simulink model "controlador_discreto"  (R2023b)
settings: Solver=FixedStepAuto  StartTime=0.0  StopTime=25  FixedStep=0.001  RelTol=1e-3
undefined symbols (not defined in the file): b_cx, b_cy, b_hb, b_hEb, b_hwu, b_t, b_tb, b_tw, bh_eq, bh_eq_prima, bt_eq, CI, ddx_t_lim, ddy_h_lim, DiscIntNeverNeededParam, dx_t_lim, dy_h_lim, g, H_c, H_SS, i_h, i_t, Jh_eq, Jh_eq_aux, Jt_eq, K_cy, K_hwu, K_tw, Kd_h, Kd_t, Ki_h, Ki_t, Kp_h, Kp_t, L_h0, M_s, m_t, r_hd, r_td, T_hb_max, T_hEb_max, T_hm_max, T_s1, T_s2, T_tb_max, T_tm_max, tau_hm, tau_tm, W_c, x_t_lim, y_c, y_h_lim, Y_t0
libraries: simulink x19, sldrtlib x1, simulink_extras x1
(part 2 of 2)

== stateflow chart controlador_discreto/Nivel 1 ==
  state Toma_carga_manual [commented out]
  state Mapeo_entradas_digitales
    accion_muelle = inputs(1);
    n_muelle = inputs(2);
    p_ini = inputs(3);
    p_fin = inputs(4);
  state Accion_carga_automatico
    state Precalculos
      % Calculos para realizar las maniobras pertinentes
      y_max = max(y_c(1:p_fin));
      %CI(3) = y_max;
      v_act = 10
    state Prueba
      carro_cons = [0 0]
      izaje_cons = [0 0]
      [carro_cons, izaje_cons] = consigna_en_muelle(T_s1, W_c, set_param_lim, n_muelle, y_max , 0, H_SS, 0, 0)
    state Toma_carga_muelle_automatico
      % Se toma carga desde posicion en muelle y se lleva al barco
      % -------------
      entry:
      [carro_cons, izaje_cons] = consigna_en_muelle(T_s1, W_c, set_param_lim, n_muelle, y_max , 0, H_SS, 0, 0);
      idx_t = 1; idx_h = 1;
      flag = 1; % CAMBIAR !!!!
      % -------------
      during:
      % Carro
      x_t = carro_cons(idx_t, 1);
      dx_t = carro_cons(idx_t, 2);
      % Izaje
      y_h = izaje_cons(idx_h, 1);
      dy_h = izaje_cons(idx_h, 2);
      if idx_t  ~=  length(carro_cons)
      idx_t = idx_t + 1;
      end
      if idx_h  ~=  length(izaje_cons)
      idx_h = idx_h + 1;
      end
      if idx_t == length(carro_cons) && idx_h == length(izaje_cons)
      flag = 1;
      end
    state Deja_carga_barco [commented out]
      % Se entra con v_t y deja carga en barco
      % -------------
      entry:
      %[carro_cons, izaje_cons] = consigna_en_barco(T_s1, W_c, H_c, y_c, set_param_lim, p_ini, p_fin, H_SS, 0, 0, 1);
      [carro_cons, izaje_cons] = consigna_en_barco(T_s1, W_c, H_c, [1 2 3], set_param_lim, 0, 1, 0.5, 0, 0, 1);
      idx_t = 1; idx_h = 1;
      flag = 0;
      % -------------
      during:
      % Carro
      x_t = carro_cons(idx_t, 1);
      dx_t = carro_cons(idx_t, 2);
      % Izaje
      y_h = izaje_cons(idx_h, 1);
      dy_h = izaje_cons(idx_h, 2);
      if idx_t  ~=  length(carro_cons)
      idx_t = idx_t + 1;
      end
      if idx_h  ~=  length(izaje_cons)
      idx_h = idx_h + 1;
      end
      if idx_t == length(carro_cons) && idx_h == length(izaje_cons)
      flag = 1;
      end
    (default) -> Precalculos
    Toma_carga_muelle_automatico -> Prueba : [flag == 1]
    Precalculos -> Toma_carga_muelle_automatico : [v_act == 10]
    Toma_carga_muelle_automatico -> Deja_carga_barco [commented out] : [flag == 1]
        | {
        | carro_cons = [0 0],
        | izaje_cons = [0 0]
        | }
  state IDLE
    entry:
    set_param_lim = [dx_t_lim ddx_t_lim dy_h_lim(1) ddy_h_lim];
    altura_izaje = 15;
    v_act = 0;
  state Deja_carga_muelle_automatico
    % Se deja carga en el muelle (especificando numero de muelle), entrando al mismo a velocidad v_act de carro
    % ------
    entry:
    [carro_cons, izaje_cons] = consigna_en_muelle(T_s1, W_c, set_param_lim, n_muelle, altura_izaje, 1, H_SS, v_act);
    idx_t = 1; idx_h = 1;
    flag = 0;
    % -------
    during:
    % Carro
    x_t = carro_cons(idx_t, 1);
    dx_t = carro_cons(idx_t, 2);
    % Izaje
    y_h = izaje_cons(idx_h, 1);
    dy_h = izaje_cons(idx_h, 2);
    if idx_t  ~=  length(carro_cons)
    idx_t = idx_t + 1;
    end
    if idx_h  ~=  length(izaje_cons)
    idx_h = idx_h + 1;
    end
    if idx_t == length(carro_cons) && idx_h == length(izaje_cons)
    flag = 1;
    end
  (default) -> Mapeo_entradas_digitales
  Mapeo_entradas_digitales -> IDLE
  IDLE -> Accion_carga_automatico [order 1] : [accion_muelle == 0]
  IDLE -> Deja_carga_muelle_automatico [order 2] : [accion_muelle == 1]
  data: inputs input size=4; T_s1 parameter; carro_cons local size=[10000; 10000] =[CI(1) CI(2)]; izaje_cons local size=[10000; 10000] =[CI(3) CI(4)]; W_c parameter; ddx_t_lim parameter; ddy_h_lim parameter; dx_t_lim parameter; dy_h_lim parameter; H_SS parameter; v_act local; set_param_lim local; n_muelle local; altura_izaje local; accion_muelle local; flag local; idx_h local; idx_t local; dx_t output size=1 =CI(2); dy_h output size=1 =CI(4); x_t output size=1 =CI(1); y_h output size=1 =CI(3); CI parameter; T_s2 parameter; t_i local; t_c local; clock input; H_c parameter; p_ini local; p_fin local; y_c parameter; v_t local; y_max local
